simulink model "PID_identification2"  (R2015a)
settings: Solver=ode45  SolverMode=SingleTasking  StartTime=0.0  StopTime=139  RelTol=1e-3
libraries: simulink x4
settings Model: CovMetricSettings=dwe  CovHtmlReporting=off  covSaveCumulativeToWorkspaceVar=off  CovSaveSingleToWorkspaceVar=off  CovExternalEMLEnable=on  Creator=DwigHT  LastModifiedBy=DwigHT
settings DataIOCC: LimitDataPoints=off  SaveFormat=Dataset  ReturnWorkspaceOutputs=on
settings DebuggingCC: UnconnectedInputMsg=none  UnconnectedOutputMsg=none  UnconnectedLineMsg=none  SFUnexpectedBacktrackingDiag=error  SFNoUnconditionalDefaultTransitionDiag=error
settings HardwareCC: ProdBitPerPointer=64  ProdLargestAtomicFloat=Float  ProdIntDivRoundTo=Zero  ProdEndianess=LittleEndian  ProdHWDeviceType=Specified
settings ModelReferenceCC: PropagateSignalLabelsOutOfModel=on
settings SFSimCC: SimUseLocalCustomCode=on
settings RTWCC: RTWUseLocalCustomCode=on
settings GRTTargetCC: TargetLangStandard=C99 (ISO)

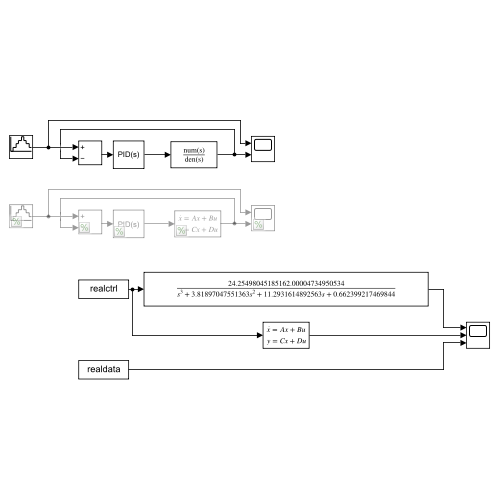
[thumbnail: Simulink's stored preview of the top-level diagram]
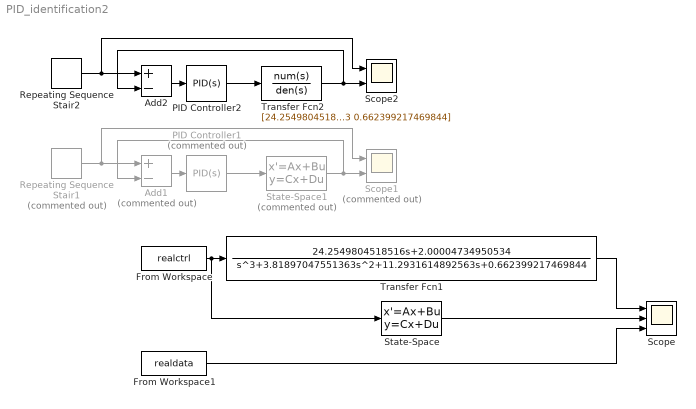
== system PID_identification2 ==
  Add1 : Sum  Commented=on  Inputs=+-
  Add2 : Sum  Inputs=+-
  From Workspace : FromWorkspace  VariableName=realctrl
  From Workspace1 : FromWorkspace  VariableName=realdata
  PID Controller1 : simulink/Continuous/PID Controller  Commented=on  Controller=PID  Form=Parallel  TimeDomain=Continuous-time  SampleTime=-1  IntegratorMethod=Forward Euler  ControllerParametersSource=internal  P=1  I=1  D=1  N=1  UseFilter=on  InitialConditionSource=internal  InitialConditionForIntegrator=0  InitialConditionForFilter=0  DifferentiatorICPrevScaledInput=0  ExternalReset=none  TrackingMode=off  Kt=1  LimitOutput=off  UpperSaturationLimit=inf  LowerSaturationLimit=-inf  LinearizeAsGain=on  AntiWindupMode=none  Kb=1  POutMin=[]  POutMax=[]  IOutMin=[]  IOutMax=[]  DOutMin=[]  DOutMax=[]  NOutMin=[]  NOutMax=[]  SumOutMin=[]  SumOutMax=[]  SaturationOutMin=[]  SaturationOutMax=[]  PParamMin=[]  PParamMax=[]  IParamMin=[]  IParamMax=[]  DParamMin=[]  DParamMax=[]  NParamMin=[]  NParamMax=[]  KbParamMin=[]  KbParamMax=[]  KtParamMin=[]  KtParamMax=[]  KbOutMin=[]  KbOutMax=[]  KtOutMin=[]  KtOutMax=[]  IntegratorOutMin=[]  IntegratorOutMax=[]  FilterOutMin=[]  FilterOutMax=[]  SumI1OutMin=[]  SumI1OutMax=[]  SumI2OutMin=[]  SumI2OutMax=[]  SumI3OutMin=[]  SumI3OutMax=[]  SumDOutMin=[]  SumDOutMax=[]  DifferentiatorOutMin=[]  DifferentiatorOutMax=[]  IntegratorContinuousStateAttributes=''  IntegratorStateMustResolveToSignalObject=off  IntegratorRTWStateStorageClass=Auto  FilterContinuousStateAttributes=''  FilterStateMustResolveToSignalObject=off  FilterRTWStateStorageClass=Auto
  PID Controller2 : simulink/Continuous/PID Controller  Controller=PID  Form=Parallel  TimeDomain=Continuous-time  SampleTime=-1  IntegratorMethod=Forward Euler  ControllerParametersSource=internal  P=1  I=1  D=1  N=1  UseFilter=on  InitialConditionSource=internal  InitialConditionForIntegrator=0  InitialConditionForFilter=0  DifferentiatorICPrevScaledInput=0  ExternalReset=none  TrackingMode=off  Kt=1  LimitOutput=off  UpperSaturationLimit=inf  LowerSaturationLimit=-inf  LinearizeAsGain=on  AntiWindupMode=none  Kb=1  POutMin=[]  POutMax=[]  IOutMin=[]  IOutMax=[]  DOutMin=[]  DOutMax=[]  NOutMin=[]  NOutMax=[]  SumOutMin=[]  SumOutMax=[]  SaturationOutMin=[]  SaturationOutMax=[]  PParamMin=[]  PParamMax=[]  IParamMin=[]  IParamMax=[]  DParamMin=[]  DParamMax=[]  NParamMin=[]  NParamMax=[]  KbParamMin=[]  KbParamMax=[]  KtParamMin=[]  KtParamMax=[]  KbOutMin=[]  KbOutMax=[]  KtOutMin=[]  KtOutMax=[]  IntegratorOutMin=[]  IntegratorOutMax=[]  FilterOutMin=[]  FilterOutMax=[]  SumI1OutMin=[]  SumI1OutMax=[]  SumI2OutMin=[]  SumI2OutMax=[]  SumI3OutMin=[]  SumI3OutMax=[]  SumDOutMin=[]  SumDOutMax=[]  DifferentiatorOutMin=[]  DifferentiatorOutMax=[]  IntegratorContinuousStateAttributes=''  IntegratorStateMustResolveToSignalObject=off  IntegratorRTWStateStorageClass=Auto  FilterContinuousStateAttributes=''  FilterStateMustResolveToSignalObject=off  FilterRTWStateStorageClass=Auto
  Repeating Sequence Stair1 : simulink/Sources/Repeating Sequence Stair  Commented=on  OutValues=[0 50 100 150 200 150 100 50].'  tsamp=10  OutMin=[]  OutMax=[]  OutDataTypeStr=double  OutputDataTypeScalingMode=double  OutDataType=fixdt(0,8)  ConRadixGroup=Best Precision: Vector-wise  OutScaling=2^-12
  Repeating Sequence Stair2 : simulink/Sources/Repeating Sequence Stair  OutValues=[0 50 100 150 200 150 100 50].'  tsamp=10  OutMin=[]  OutMax=[]  OutDataTypeStr=double  OutputDataTypeScalingMode=double  OutDataType=fixdt(0,8)  ConRadixGroup=Best Precision: Vector-wise  OutScaling=2^-12
  Scope : Scope  NumInputPorts=3
      settings: TimeRange=auto  MaxDataPoints=5000  SaveToWorkspace=off  SaveName=ScopeData  YMin=-70.95875~-5~-5  YMax=325.09114~5~5  SampleTime=-1
  Scope1 : Scope  Commented=on  NumInputPorts=2
      settings: TimeRange=auto  MaxDataPoints=5000  SaveToWorkspace=off  YMin=-92717812636169899244857306144429302039534528938674381880076001775071661168457031381336886575931848855199215905328537264302988329894979122797898042187515413119133838557705542583154091305069429572148315664009088740452430779394652935133285511544399682740121975956107509422192032945050682658651337501298820907008.00000~-5  YMax=49218839720335017302619930094552326426152078761959868996293440079387663904843679041741564748800837477295537476208663880789442735120258938551150781383339642910239692214264854455933004655876280314888480102361503091572419546960066851369316493435345242815520056344733166856019087265009895563869980508202555408384.00000~5  SampleTime=-1
  Scope2 : Scope  NumInputPorts=2
      settings: TimeRange=auto  MaxDataPoints=5000  SaveToWorkspace=off  SaveName=ScopeData2  YMin=-38.0762~-5  YMax=238.10492~5  SampleTime=-1
  State-Space : StateSpace  A=|  B=|  C="[506.6935  -28.5861   20.0306]"  D=0  X0=0
      A=|
      | [-0.1138    2.9137   -1.5672;
      |    -4.9175   -7.2086    8.0717;
      |     1.4734   -0.1860   -1.7556]
      B=|
      | [-0.0193;
      |     0.0886;
      |    -0.0121]
  State-Space1 : StateSpace  Commented=on  A=|  B=|  C="[506.6935  -28.5861   20.0306]"  D=0  X0=0
      A=|
      | [-0.1138    2.9137   -1.5672;
      |    -4.9175   -7.2086    8.0717;
      |     1.4734   -0.1860   -1.7556]
      B=|
      | [-0.0193;
      |     0.0886;
      |    -0.0121]
  Transfer Fcn1 : TransferFcn  Numerator="[24.2549804518516\t2.00004734950534]"  Denominator=[1 3.81897047551363 11.2931614892563 0.662399217469844]
  Transfer Fcn2 : TransferFcn  Numerator="[24.2549804518516\t2.00004734950534]"  Denominator=[1 3.81897047551363 11.2931614892563 0.662399217469844]
  wires:
  Repeating Sequence Stair1/1 -> Scope1/1, Add1/1
  State-Space1/1 -> Scope1/2, Add1/2
  PID Controller1/1 -> State-Space1/1
  Add1/1 -> PID Controller1/1
  From Workspace/1 -> State-Space/1, Transfer Fcn1/1
  Transfer Fcn1/1 -> Scope/1
  From Workspace1/1 -> Scope/3
  State-Space/1 -> Scope/2
  Add2/1 -> PID Controller2/1
  PID Controller2/1 -> Transfer Fcn2/1
  Transfer Fcn2/1 -> Add2/2, Scope2/2
  Repeating Sequence Stair2/1 -> Add2/1, Scope2/1
